simulink model "Solar_Tracker_Model_Dual_axis"  (R2024a)
settings: Solver=ode45  StartTime=0.0  StopTime=24  MaxStep=0.01  RelTol=1e-3
PreLoadFcn:
  | addpath(fullfile('WormAndGearConstraintSupport','Data'));
  | addpath(fullfile('WormAndGearConstraintSupport','Scripts'));
model workspace: external: MATLAB File WormAndGearConstraintParameters.m (data not in the file)
undefined symbols (not defined in the file): X, Y, Z
libraries: fl_lib x42, nesl_utility x18, WormAndGearConstraintLibrary x18, fl_ps_legacy_lib x17, sm_lib x9, ee_lib x4, simulink x2, SignalEditorBlockLib x2
(part 1 of 2)
CloseFcn:
  | rmpath(fullfile('WormAndGearConstraintSupport','Data'));
  | rmpath(fullfile('WormAndGearConstraintSupport','Scripts'));
Description:
  | Accurately sets up the solar panel according to the Sun's position
  | Project Name: Solar Tracker
  | Author: Kanak Sharma
  | Email: kanak.sharma1031@gmail.com
  | Date: 2024-06-25
  | License: This project is licensed under the MIT License - see the LICENSE file for details.
settings Model: Creator=The MathWorks, Inc.  LastModifiedBy=AADIL MALIK
settings SolverCC: AlgebraicLoopSolver=TrustRegion
settings DataIOCC: ReturnWorkspaceOutputs=off
settings OptimizationCC: ReuseModelBlockBuffer=off
settings DebuggingCC: UnconnectedInputMsg=warning  UnconnectedOutputMsg=warning  UnconnectedLineMsg=warning  SubsystemReferenceDiagnosticForUnitTest=warning  ArithmeticOperatorsInVariantConditions=warning
settings ModelReferenceCC: EnableRefExpFcnMdlSchedulingChecks=on
settings SFSimCC: SimUseLocalCustomCode=off  CustomCodeUndefinedFunction=UseInterfaceOnly
settings RTWCC: RTWUseLocalCustomCode=off  GPUComputeCapability=3.5
settings CodeAppCC: StateflowObjectComments=on
settings ConfigComp: CovMetricSettings=dswe
settings SimscapeCC: ExplicitSolverDiagnosticOptions=none  SimscapeNormalizeSystem=off  SimscapeNominalValues="[{\"value\":\"10\",\"unit\":\"V\"},{\"value\":\"1\",\"unit\":\"A\"},{\"value\":\"10\",\"unit\":\"N*m\"},{\"value\":\"10\",\"unit\":\"bar\"},{\"value\":\"100\",\"unit\":\"kJ/kg\"},{\"value\":\"1\",\"unit\":\"kW\"},{\"value\":\"300\",\"unit\":\"K\"},{\"value\":\"100\",\"unit\":\"cm^3/s\"},{\"value\":\"1\",\"unit\":\"kN\"},{\"value\":\"1\",\"unit\":\"g/cm^3\"},{\"value\":\"1\",\"unit\":\"l\"},{\"value\":\"1\",\"unit\":\"cm^2\"},{\"value\":\"60\",\"unit\":\"Hz\"}]"  SimscapeLogType=all  SimscapeLogSimulationStatistics=on  SimscapeLogName=simlogWormAndGearConstraint
settings DiagnosticsConfigSet: SimMechanicsUnconnectedFramePorts=none
settings ExplorerConfigSet: InternalSimMechanicsExplorerSettings="<ExplorerConfiguration><canonicalview>default</canonicalview><AnimationSetting><BasePlaybackSpeed>1.0</BasePlaybackSpeed><PlaybackSpeedFactor>1.0</PlaybackSpeedFactor></AnimationSetting><TilePanel><TileInfo><Tiles Columns=\"1\" Count=\"2\" Rows=\"2\"><Column Left=\"2\" Weight=\"1\"/><Column Left=\"959\" Weight=\"0.5003\"/><Row Top=\"2\" Weight=\"0.499\"/><Row Top=\"438\" Weight=\"0.501\"/><Row Top=\"875\"/><Tile Height=\"1\" Width=\"1\" X=\"0\" Y=\"0\"/><Tile Height=\"1\" Width=\"1\" X=\"0\" Y=\"1\"/></Tiles></TileInfo><SceneInfo><SceneViewer><BGColor><R>0.60000002384185791</R><G>0.60000002384185791</G><B>0.60000002384185791</B></BGColor><Camera><DoPerspective>off</DoPerspective><Position><X>1.5722270375482781</X><Y>0.036026125950558319</Y><Z>2.5132450829803226</Z></Position><Center><X>0.030597625568977493</X><Y>1.5776555379298589</Y><Z>0.97161567100102131</Z></Center><Up><X>-0.40824829046386307</X><Y>0.40824829046386307</Y><Z>0.81649658092772615</Z></Up><ViewLimDist>1</ViewLimDist><YLim>1.5517509961128235</YLim><XLim>3.445105256006924</XLim></Camera></SceneViewer><SceneViewer><BGColor><R>0.60000002384185791</R><G>0.60000002384185791</G><B>0.60000002384185791</B></BGColor><Camera><DoPerspective>on</DoPerspective><Position><X>0.052898448769590822</X><Y>3.2815089600888423</Y><Z>1.0106868675116196</Z></Position><Center><X>-0.01109217435380673</X><Y>3.0487464713239714</Y><Z>0.94979470185928261</Z></Center><Up><X>-0.054323829999052796</X><Y>-0.23871114009518463</Y><Z>0.96956996296744424</Z></Up><ViewLimDist>1</ViewLimDist><YLim>0.46630765815499858</YLim><XLim>1.0328496727358381</XLim></Camera></SceneViewer></SceneInfo></TilePanel><MechEditorPanel><Cameras><Camera><Id>Camera1</Id><Value><Name>Slew Drive View</Name><NativeCamera><PositionKeyframeSet><Keyframe><Time>+0.0000000000000000e+00</Time><Value><X>+5.2898448769590822e-02</X><Y>+3.2815089600888423e+00</Y><Z>+1.0106868675116196e+00</Z></Value></Keyframe></PositionKeyframeSet><CenterKeyframeSet><Keyframe><Time>+0.0000000000000000e+00</Time><Value><X>-1.1092174353806730e-02</X><Y>+3.0487464713239714e+00</Y><Z>+9.4979470185928261e-01</Z></Value></Keyframe></CenterKeyframeSet><UpVectorKeyframeSet><Keyframe><Time>+0.0000000000000000e+00</Time><Value><X>-5.4323829999052796e-02</X><Y>-2.3871114009518463e-01</Y><Z>+9.6956996296744424e-01</Z></Value></Keyframe></UpVectorKeyframeSet></NativeCamera></Value></Camera></Cameras><GfxPanelCameraMap><MapElement CameraMLId=\"Camera1\" GfxPanelIndex=\"1\"/></GfxPanelCameraMap><VideoCreator><PlaybackSpeedRatio>1.0</PlaybackSpeedRatio><FrameRate>30</FrameRate><VideoFormat>Motion JPEG AVI</VideoFormat><FrameSize>auto</FrameSize></VideoCreator></MechEditorPanel></ExplorerConfiguration>"

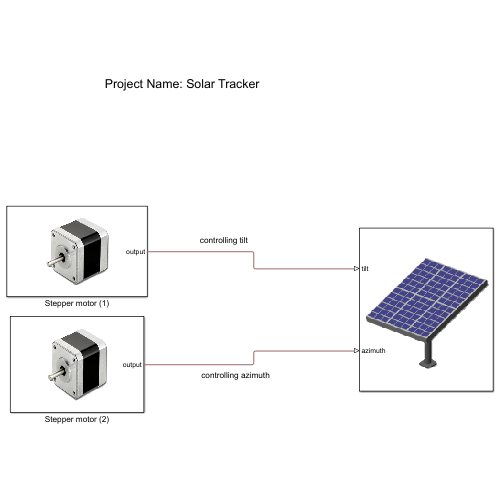
[thumbnail: Simulink's stored preview of the top-level diagram]
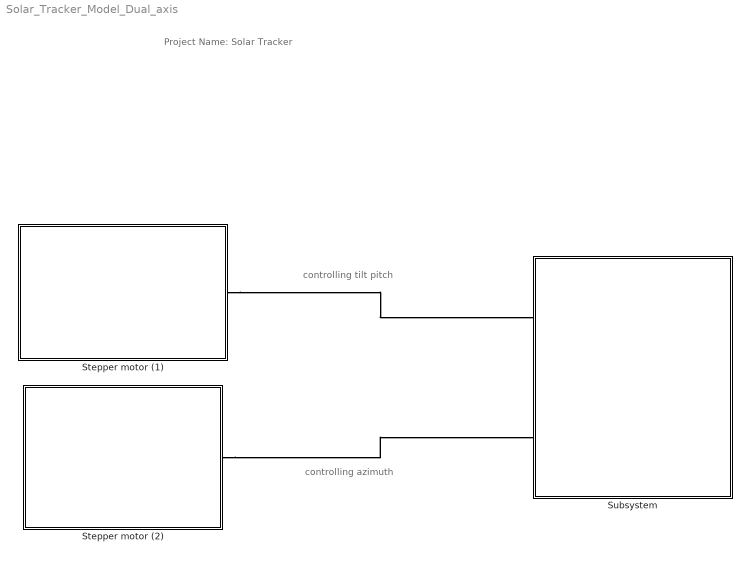
== system Solar_Tracker_Model_Dual_axis ==
  note: controlling azimuth
  note: controlling tilt pitch
  note: Project Name: Solar Tracker
  Stepper motor (1) : Subsystem
      mask Display: image('stepper_motor.jpg');
  Stepper motor (2) : Subsystem
      mask Display: image('stepper_motor.jpg');
  Subsystem : Subsystem
      mask Display: image('SolarTracker.png');
  connections:
  Stepper motor (1)/RConn1 -- Subsystem/LConn1
  Stepper motor (2)/RConn1 -- Subsystem/LConn2

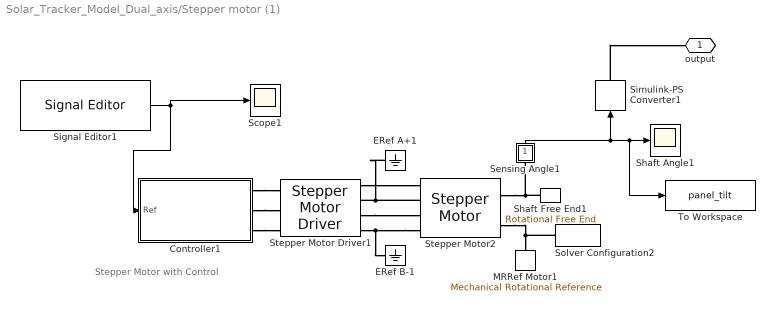
== system Solar_Tracker_Model_Dual_axis/Stepper motor (1) ==
  note: Stepper Motor with Control
  Controller1 : Subsystem  Variant=on  VariantControlMode=label  LabelModeActiveChoice=Position
      settings: AttributesFormatString=%<BlockChoice>
  ERef A+1 : fl_lib/Electrical/Electrical Elements/Electrical Reference
  ERef B-1 : fl_lib/Electrical/Electrical Elements/Electrical Reference
  MRRef Motor1 : fl_lib/Mechanical/Rotational Elements/Mechanical Rotational Reference
  Scope1 : Scope
  Sensing Angle1 : Subsystem
      mask Display: disp('a')
  Shaft Angle1 : Scope
  Shaft Free End1 : fl_lib/Mechanical/Rotational Elements/Rotational Free End  w_specify=off  w_priority=None  w=0 rad/s  w_nominal_specify=off  w_nominal_value=1  w_nominal_unit=rad/s
  Signal Editor1 : SignalEditorBlockLib/Signal Editor  FileName=elevation_signal_data.mat  ActiveScenario=dataset  ActiveSignal=elevation_signal_data  IsBus=off  OutputBusObjectStr=Bus: BusObject  SampleTime=0  Interpolate=off  ZeroCross=off  OutputAfterFinalValue=Setting to zero  Unit=inherit  PreserveSignalName=on  ApplySigPropsToAllScenarios=on  ApplySigPropsToAllSignals=off
  Simulink-PS Converter1 : nesl_utility/Simulink-PS Converter  PhysicalDomain=network_engine_domain  SubClassName=ps_input  LeftPortType=input  RightPortType=output  PseudoPeriodic=off  Frequencies=[]  NoiseDistribution=none  NoiseParameters=[]  Unit=deg  AffineConversion=off  FilteringAndDerivatives=filter  SimscapeFilterOrder=2  InputFilterTimeConstant=yawsignal.t_c  UdotUserProvided=1
  Solver Configuration2 : nesl_utility/Solver Configuration  PhysicalDomain=network_engine_domain  SubClassName=solver  LeftPortType=input  RightPortType=generic  Tones=[]  Harmonics=[]  SimulateNoise=off  Profile=off  UseLocalSampling=off  EnableSwitchedLinearOptims=on  FrequencyDomain=off  UseCCode=off  RelTol=0.001  AbsTol=1e-06  MinStep=1e-09  ToWorkspace=off  RevertToSquareIcSolve=off  NumHomotopyIterations=100  PhasorMode=off  PhasorModeNumHarmonics=1  ConsistencySolver=NEWTON_FTOL  IndexReductionMethod=DerivativeReplacement  DoDC=off  ResidualTolerance=1e-9  ConsistencyTolSource=GLOBAL  ConsistencyAbsTol=0.001  ConsistencyRelTol=0.001  ConsistencyTolFactor=0.001  UseLocalSolver=off  LocalSolverChoice=NE_BACKWARD_EULER_ADVANCER  ResolveIndetEquations=on  FunctionEvalNumThread=1  LocalSolverSampleTime=.001  DoFixedCost=off  MaxNonlinIter=3  MaxModeIter=2  ComputeImpulses=off  ImpulseIterations=2  LinearAlgebra=auto  LinearAlgebraNumThread=0  EquationFormulation=NE_TIME_EF  DelaysMemoryBudget=1024  AutomaticFiltering=on  FilteringTimeConstant=0.001  PartitionStorageMethod=AS_NEEDED  PartitionMemoryBudget=1024  PartitionMethod=FAST  MultibodyUseLocalSolver=off  MultibodyLocalSolverChoice=ODE1  MultibodyLocalSolverSampleTime=0.001
  Stepper Motor Driver1 : ee_lib/Electromechanical/Reluctance & Stepper/Stepper Motor Driver  step_or_av=1  step_rate_per_volt=10 Hz/V  Venable=2.5 V  Vreverse=2.5 V  supply_ports=ee.enum.supply_ports.hidesupply  Vm=5 V  Vsupply=10 V  half_stepping=0  stepping_mode=ee.enum.electromech.steppingMode.fullStep  numMicroSteps=4  Im=1.2 A
      settings: InternalSimscapePortConfiguration="{\"Bottom\":[],\"Left\":[{\"id\":\"ENA\",\"label\":\"ENA\",\"type\":\"foundation.electrical.electrical\"},{\"id\":\"REF\",\"label\":\"REF\",\"type\":\"foundation.electrical.electrical\"},{\"id\":\"REV\",\"label\":\"REV\",\"type\":\"foundation.electrical.electrical\"}],\"Right\":[{\"id\":\"pA\",\"label\":\"A+\",\"type\":\"foundation.electrical.electrical\"},{\"id\":\"nA\",\"label\":\"A-\",\"type\":\"foundation.electrical.electrical\"},{\"id\":\"pB\",\"label\":\"B+\",\"type\":\"foundation.electrical.electrical\"},{\"id\":\"nB\",\"label\":\"B-\",\"type\":\"foundation.electrical.electrical\"}],\"Top\":[]}"
  Stepper Motor2 : ee_lib/Electromechanical/Reluctance & Stepper/Stepper Motor  step_or_av=1  Ra=0.55 Ohm  La=0.0015 H  Km=0.19 N*m/A  Td=0 N*m  Rm=Inf Ohm  w_vec=[ 0 1000 3e+3 ] rpm  T_vec=[ 2 2 1 ] N*m  assert_if_slipping=0  J_total=1e-4 kg*m^2  max_step_rate=10 Hz  Step=1.8 deg  J=4.5e-05 kg*m^2  B=1e-02 N*m/(rad/s)  speed0=0 rpm  theta0=0 deg  alpha=[.00393, .00393] 1/K  Tmeas=25 degC  Tmeas2=125 degC  T_vec2=[1.7, 1.7, .85] N*m  half_stepping=ee.enum.electromech.steppingModeAveraged.fullStep  thermal_masses=[100, 100] J/K  initial_temperatures=[25, 25] degC  rotor_thermal_mass=50 J/K  rotor_initial_temperature=25 degC  Rm_percent_rotor=90
      settings: InternalSimscapePortConfiguration="{\"Bottom\":[],\"Left\":[{\"id\":\"pA\",\"label\":\"A+\",\"type\":\"foundation.electrical.electrical\"},{\"id\":\"nA\",\"label\":\"A-\",\"type\":\"foundation.electrical.electrical\"},{\"id\":\"pB\",\"label\":\"B+\",\"type\":\"foundation.electrical.electrical\"},{\"id\":\"nB\",\"label\":\"B-\",\"type\":\"foundation.electrical.electrical\"}],\"Right\":[{\"id\":\"R\",\"label\":\"R\",\"type\":\"foundation.mechanical.rotational.rotational\"},{\"id\":\"C\",\"label\":\"C\",\"type\":\"foundation.mechanical.rotational.rotational\"}],\"Top\":[]}"
  To Workspace : ToWorkspace  VariableName=panel_tilt  SampleTime=-1
  output : PMIOPort  Side=Right
  wires:
  Signal Editor1/1 -> Scope1/1, Controller1/1(Ref)
  Sensing Angle1/1(theta) -> Simulink-PS Converter1/1, To Workspace/1, Shaft Angle1/1
  connections:
  Stepper Motor2/LConn4 -- Stepper Motor Driver1/RConn4 -- ERef B-1/LConn1
  Stepper Motor Driver1/RConn3 -- Stepper Motor2/LConn3
  Solver Configuration2/RConn1 -- Stepper Motor2/RConn2 -- MRRef Motor1/LConn1
  Shaft Free End1/LConn1 -- Stepper Motor2/RConn1 -- Sensing Angle1/LConn1
  Controller1/RConn3 -- Stepper Motor Driver1/LConn3
  Controller1/RConn1 -- Stepper Motor Driver1/LConn1
  Controller1/RConn2 -- Stepper Motor Driver1/LConn2
  Simulink-PS Converter1/RConn1 -- output/RConn1
  ERef A+1/LConn1 -- Stepper Motor2/LConn2 -- Stepper Motor Driver1/RConn2
  Stepper Motor Driver1/RConn1 -- Stepper Motor2/LConn1

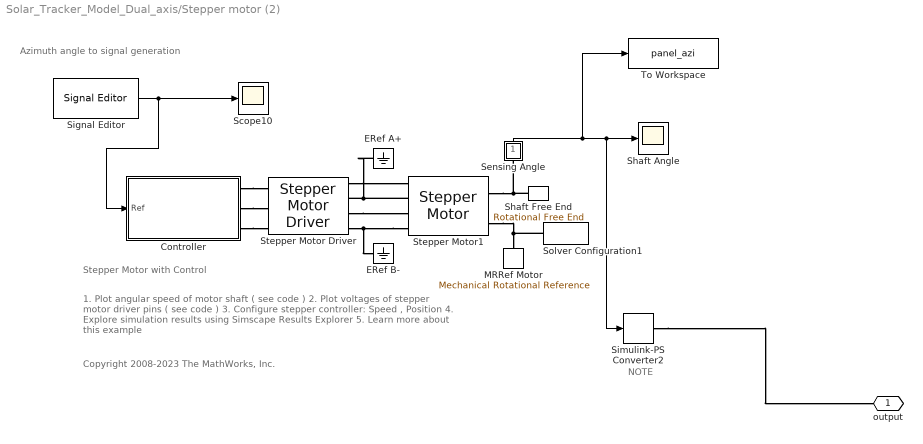
== system Solar_Tracker_Model_Dual_axis/Stepper motor (2) ==
  note: NOTE
  note: Stepper Motor with Control
  note: 1. Plot angular speed of motor shaft ( see code )
      | 2. Plot voltages of stepper motor driver pins ( see code )
      | 3. Configure stepper controller: Speed , Position
      | 4. Explore simulation results using Simscape Results Explorer
      | 5. Learn more about this example
  note: Azimuth angle to signal generation
  note: Copyright 2008-2023 The MathWorks, Inc.
  Controller : Subsystem  Variant=on  VariantControlMode=label  LabelModeActiveChoice=Position
      settings: AttributesFormatString=%<BlockChoice>
  ERef A+ : fl_lib/Electrical/Electrical Elements/Electrical Reference
  ERef B- : fl_lib/Electrical/Electrical Elements/Electrical Reference
  MRRef Motor : fl_lib/Mechanical/Rotational Elements/Mechanical Rotational Reference
  Scope10 : Scope
  Sensing Angle : Subsystem
      mask Display: disp('a')
  Shaft Angle : Scope
  Shaft Free End : fl_lib/Mechanical/Rotational Elements/Rotational Free End  w_specify=off  w_priority=None  w=0 rad/s  w_nominal_specify=off  w_nominal_value=1  w_nominal_unit=rad/s
  Signal Editor : SignalEditorBlockLib/Signal Editor  FileName=azimuth_signal_data.mat  ActiveScenario=dataset  ActiveSignal=azimuth_signal_data  IsBus=off  OutputBusObjectStr=Bus: BusObject  SampleTime=0  Interpolate=off  ZeroCross=off  OutputAfterFinalValue=Setting to zero  Unit=inherit  PreserveSignalName=on  ApplySigPropsToAllScenarios=on  ApplySigPropsToAllSignals=off
  Simulink-PS Converter2 : nesl_utility/Simulink-PS Converter  PhysicalDomain=network_engine_domain  SubClassName=ps_input  LeftPortType=input  RightPortType=output  PseudoPeriodic=off  Frequencies=[]  NoiseDistribution=none  NoiseParameters=[]  Unit=deg  AffineConversion=off  FilteringAndDerivatives=filter  SimscapeFilterOrder=2  InputFilterTimeConstant=yawsignal.t_c  UdotUserProvided=1
  Solver Configuration1 : nesl_utility/Solver Configuration  PhysicalDomain=network_engine_domain  SubClassName=solver  LeftPortType=input  RightPortType=generic  Tones=[]  Harmonics=[]  SimulateNoise=off  Profile=off  UseLocalSampling=off  EnableSwitchedLinearOptims=on  FrequencyDomain=off  UseCCode=off  RelTol=0.001  AbsTol=1e-06  MinStep=1e-09  ToWorkspace=off  RevertToSquareIcSolve=off  NumHomotopyIterations=100  PhasorMode=off  PhasorModeNumHarmonics=1  ConsistencySolver=NEWTON_FTOL  IndexReductionMethod=DerivativeReplacement  DoDC=off  ResidualTolerance=1e-9  ConsistencyTolSource=GLOBAL  ConsistencyAbsTol=0.001  ConsistencyRelTol=0.001  ConsistencyTolFactor=0.001  UseLocalSolver=off  LocalSolverChoice=NE_BACKWARD_EULER_ADVANCER  ResolveIndetEquations=on  FunctionEvalNumThread=1  LocalSolverSampleTime=.001  DoFixedCost=off  MaxNonlinIter=3  MaxModeIter=2  ComputeImpulses=off  ImpulseIterations=2  LinearAlgebra=auto  LinearAlgebraNumThread=0  EquationFormulation=NE_TIME_EF  DelaysMemoryBudget=1024  AutomaticFiltering=on  FilteringTimeConstant=0.001  PartitionStorageMethod=AS_NEEDED  PartitionMemoryBudget=1024  PartitionMethod=FAST  MultibodyUseLocalSolver=off  MultibodyLocalSolverChoice=ODE1  MultibodyLocalSolverSampleTime=0.001
  Stepper Motor Driver : ee_lib/Electromechanical/Reluctance & Stepper/Stepper Motor Driver  step_or_av=1  step_rate_per_volt=10 Hz/V  Venable=2.5 V  Vreverse=2.5 V  supply_ports=ee.enum.supply_ports.hidesupply  Vm=5 V  Vsupply=10 V  half_stepping=0  stepping_mode=ee.enum.electromech.steppingMode.fullStep  numMicroSteps=4  Im=1.2 A
      settings: InternalSimscapePortConfiguration="{\"Bottom\":[],\"Left\":[{\"id\":\"ENA\",\"label\":\"ENA\",\"type\":\"foundation.electrical.electrical\"},{\"id\":\"REF\",\"label\":\"REF\",\"type\":\"foundation.electrical.electrical\"},{\"id\":\"REV\",\"label\":\"REV\",\"type\":\"foundation.electrical.electrical\"}],\"Right\":[{\"id\":\"pA\",\"label\":\"A+\",\"type\":\"foundation.electrical.electrical\"},{\"id\":\"nA\",\"label\":\"A-\",\"type\":\"foundation.electrical.electrical\"},{\"id\":\"pB\",\"label\":\"B+\",\"type\":\"foundation.electrical.electrical\"},{\"id\":\"nB\",\"label\":\"B-\",\"type\":\"foundation.electrical.electrical\"}],\"Top\":[]}"
  Stepper Motor1 : ee_lib/Electromechanical/Reluctance & Stepper/Stepper Motor  step_or_av=1  Ra=0.55 Ohm  La=0.0015 H  Km=0.19 N*m/A  Td=0 N*m  Rm=Inf Ohm  w_vec=[ 0 1000 3e+3 ] rpm  T_vec=[ 2 2 1 ] N*m  assert_if_slipping=0  J_total=1e-4 kg*m^2  max_step_rate=10 Hz  Step=1.8 deg  J=4.5e-05 kg*m^2  B=1e-02 N*m/(rad/s)  speed0=0 rpm  theta0=0 deg  alpha=[.00393, .00393] 1/K  Tmeas=25 degC  Tmeas2=125 degC  T_vec2=[1.7, 1.7, .85] N*m  half_stepping=ee.enum.electromech.steppingModeAveraged.fullStep  thermal_masses=[100, 100] J/K  initial_temperatures=[25, 25] degC  rotor_thermal_mass=50 J/K  rotor_initial_temperature=25 degC  Rm_percent_rotor=90
      settings: InternalSimscapePortConfiguration="{\"Bottom\":[],\"Left\":[{\"id\":\"pA\",\"label\":\"A+\",\"type\":\"foundation.electrical.electrical\"},{\"id\":\"nA\",\"label\":\"A-\",\"type\":\"foundation.electrical.electrical\"},{\"id\":\"pB\",\"label\":\"B+\",\"type\":\"foundation.electrical.electrical\"},{\"id\":\"nB\",\"label\":\"B-\",\"type\":\"foundation.electrical.electrical\"}],\"Right\":[{\"id\":\"R\",\"label\":\"R\",\"type\":\"foundation.mechanical.rotational.rotational\"},{\"id\":\"C\",\"label\":\"C\",\"type\":\"foundation.mechanical.rotational.rotational\"}],\"Top\":[]}"
  To Workspace : ToWorkspace  VariableName=panel_azi  SampleTime=-1
  output : PMIOPort  Side=Right
  wires:
  Sensing Angle/1(theta) -> To Workspace/1, Simulink-PS Converter2/1, Shaft Angle/1
  Signal Editor/1 -> Controller/1(Ref), Scope10/1
  connections:
  Controller/RConn2 -- Stepper Motor Driver/LConn2
  Stepper Motor1/LConn4 -- Stepper Motor Driver/RConn4 -- ERef B-/LConn1
  Solver Configuration1/RConn1 -- Stepper Motor1/RConn2 -- MRRef Motor/LConn1
  ERef A+/LConn1 -- Stepper Motor1/LConn2 -- Stepper Motor Driver/RConn2
  Shaft Free End/LConn1 -- Stepper Motor1/RConn1 -- Sensing Angle/LConn1
  Controller/RConn1 -- Stepper Motor Driver/LConn1
  Stepper Motor Driver/RConn3 -- Stepper Motor1/LConn3
  Controller/RConn3 -- Stepper Motor Driver/LConn3
  Stepper Motor Driver/RConn1 -- Stepper Motor1/LConn1
  Simulink-PS Converter2/RConn1 -- output/RConn1

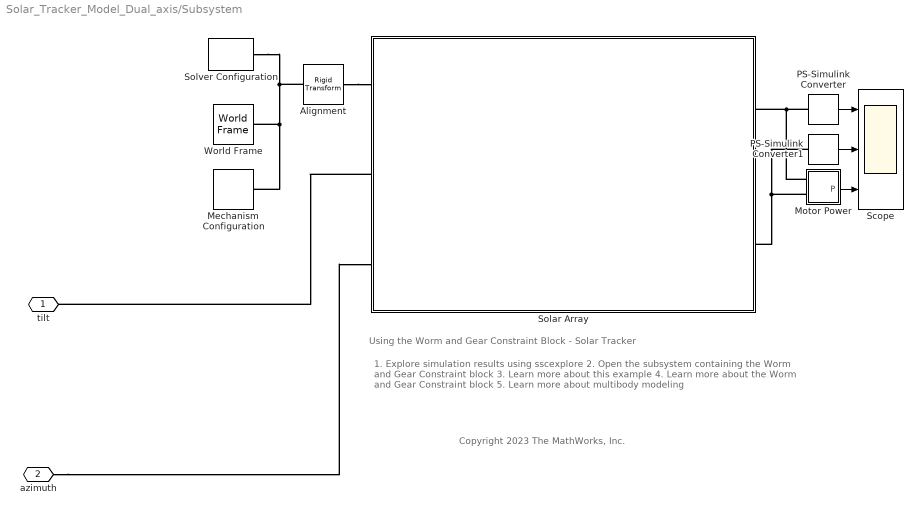
== system Solar_Tracker_Model_Dual_axis/Subsystem ==
  note: Copyright 2023 The MathWorks, Inc.
  note: Using the Worm and Gear Constraint Block - Solar Tracker
  note: 1. Explore simulation results using sscexplore
      | 2. Open the subsystem containing the Worm and Gear Constraint block
      | 3. Learn more about this example
      | 4. Learn more about the Worm and Gear Constraint block
      | 5. Learn more about multibody modeling
  Alignment : sm_lib/Frames and Transforms/Rigid Transform  RotationMethod=AlignedAxes  FollAlignAxisA=+Z  BaseAlignAxisA=+Z  FollAlignAxisB=+Y  BaseAlignAxisB=-X  RotationStandardAxis=+Z  RotationAngle=0.0  RotationAngleUnits=deg  RotationArbitraryAxis=[0 0 1]  RotationSequenceAxes=FollowerAxes  RotationSequence=XYX  RotationSequenceAngles=[0 0 0]  RotationSequenceAnglesUnits=deg  RotationMatrix=[1 0 0; 0 1 0; 0 0 1]  Quaternion=[1 0 0 0]  TranslationMethod=None  TranslationCartesianOffset=[0 0 0]  TranslationCartesianOffsetUnits=m  TranslationStandardAxis=+Z  TranslationStandardOffset=0  TranslationStandardOffsetUnits=m  TranslationROffset=0  TranslationROffsetUnits=m  TranslationThetaOffset=0  TranslationThetaOffsetUnits=deg  TranslationZOffset=0  TranslationZOffsetUnits=m
  Mechanism Configuration : sm_lib/Utilities/Mechanism Configuration  UniformGravity=Constant  GravityVector=[0 0 -9.80665]  GravityVectorUnits=m/s^2  LinearizationDelta=0.001  JointModeTransitionNonlinearIterations=2
  Motor Power : Subsystem
  PS-Simulink Converter : nesl_utility/PS-Simulink Converter  PhysicalDomain=network_engine_domain  SubClassName=ps_output  LeftPortType=input  RightPortType=output  PseudoPeriodic=off  Frequencies=[]  VectorFormat=1-D array  Unit=deg/s  AffineConversion=off
  PS-Simulink Converter1 : nesl_utility/PS-Simulink Converter  PhysicalDomain=network_engine_domain  SubClassName=ps_output  LeftPortType=input  RightPortType=output  PseudoPeriodic=off  Frequencies=[]  VectorFormat=1-D array  Unit=N*m  AffineConversion=off
  Scope : Scope  NumInputPorts=3
  Solar Array : Subsystem
      mask Display:
      | image(fullfile('WormAndGearConstraintSupport','Images','SolarArray.png'));
      | port_label('lconn',1,'W');
      | port_label('lconn',2,'yaw');
      | port_label('lconn',3,'pitch');
      | port_label('rconn',1,'wWorm');
      | port_label('rconn',2,'tWorm');
  Solver Configuration : nesl_utility/Solver Configuration  PhysicalDomain=network_engine_domain  SubClassName=solver  LeftPortType=input  RightPortType=generic  Tones=[]  Harmonics=[]  SimulateNoise=off  Profile=off  UseLocalSampling=off  EnableSwitchedLinearOptims=on  FrequencyDomain=off  UseCCode=off  RelTol=0.001  AbsTol=1e-06  MinStep=1e-09  ToWorkspace=off  RevertToSquareIcSolve=off  NumHomotopyIterations=100  PhasorMode=off  PhasorModeNumHarmonics=1  ConsistencySolver=NEWTON_FTOL  IndexReductionMethod=DerivativeReplacement  DoDC=off  ResidualTolerance=1e-09  ConsistencyTolSource=GLOBAL  ConsistencyAbsTol=0.001  ConsistencyRelTol=0.001  ConsistencyTolFactor=0.001  UseLocalSolver=off  LocalSolverChoice=NE_BACKWARD_EULER_ADVANCER  ResolveIndetEquations=on  FunctionEvalNumThread=1  LocalSolverSampleTime=0.001  DoFixedCost=off  MaxNonlinIter=3  MaxModeIter=2  ComputeImpulses=off  ImpulseIterations=2  LinearAlgebra=Sparse  LinearAlgebraNumThread=0  EquationFormulation=NE_TIME_EF  DelaysMemoryBudget=1024  AutomaticFiltering=on  FilteringTimeConstant=0.001  PartitionStorageMethod=AS_NEEDED  PartitionMemoryBudget=1024  PartitionMethod=FAST  MultibodyUseLocalSolver=off  MultibodyLocalSolverChoice=ODE1  MultibodyLocalSolverSampleTime=0.001
  World Frame : sm_lib/Frames and Transforms/World Frame
  tilt : PMIOPort  Side=Left
  azimuth : PMIOPort  Port=2  Side=Left
  wires:
  PS-Simulink Converter1/1 -> Scope/2
  Motor Power/1(P) -> Scope/3
  PS-Simulink Converter/1 -> Scope/1
  connections:
  PS-Simulink Converter/LConn1 -- Motor Power/LConn1 -- Solar Array/RConn1
  World Frame/RConn1 -- Solver Configuration/RConn1 -- Alignment/LConn1 -- Mechanism Configuration/RConn1
  Alignment/RConn1 -- Solar Array/LConn1
  PS-Simulink Converter1/LConn1 -- Motor Power/LConn2 -- Solar Array/RConn2
  azimuth/RConn1 -- Solar Array/LConn3
  Solar Array/LConn2 -- tilt/RConn1

== system Solar_Tracker_Model_Dual_axis/Stepper motor (1)/Controller1 ==
  Ref : Inport
  Position : Subsystem  VariantControl=Position
  Speed : Subsystem  VariantControl=Speed
  PWM : PMIOPort  Side=Right
  0v : PMIOPort  Port=2  Side=Right
  REV : PMIOPort  Port=3  Side=Right

== system Solar_Tracker_Model_Dual_axis/Stepper motor (1)/Sensing Angle1 ==
  MRRef : fl_lib/Mechanical/Rotational Elements/Mechanical Rotational Reference
  Motion Sensor : fl_lib/Mechanical/Mechanical Sensors/Ideal Rotational Motion Sensor  reference=foundation.enum.MeasurementReference.difference  acceleration_port=false  velocity_port=true  position_port=true  wrap_angle=simscape.enum.onoff.off  offset=0 rad
  deg : nesl_utility/PS-Simulink Converter  PhysicalDomain=network_engine_domain  SubClassName=ps_output  LeftPortType=input  RightPortType=output  PseudoPeriodic=off  Frequencies=[]  VectorFormat=1-D array  Unit=deg  AffineConversion=off
  R : PMIOPort  Side=Left
  theta : Outport  VectorParamsAs1DForOutWhenUnconnected=off
  wires:
  deg/1 -> theta/1
  connections:
  R/RConn1 -- Motion Sensor/LConn1
  Motion Sensor/RConn3 -- deg/LConn1
  MRRef/LConn1 -- Motion Sensor/RConn1

== system Solar_Tracker_Model_Dual_axis/Stepper motor (2)/Controller ==
  Ref : Inport
  Position : Subsystem  VariantControl=Position
  Speed : Subsystem  VariantControl=Speed
  PWM : PMIOPort  Side=Right
  0v : PMIOPort  Port=2  Side=Right
  REV : PMIOPort  Port=3  Side=Right

== system Solar_Tracker_Model_Dual_axis/Stepper motor (2)/Sensing Angle ==
  MRRef : fl_lib/Mechanical/Rotational Elements/Mechanical Rotational Reference
  Motion Sensor : fl_lib/Mechanical/Mechanical Sensors/Ideal Rotational Motion Sensor  reference=foundation.enum.MeasurementReference.difference  acceleration_port=false  velocity_port=true  position_port=true  wrap_angle=simscape.enum.onoff.off  offset=0 rad
  deg : nesl_utility/PS-Simulink Converter  PhysicalDomain=network_engine_domain  SubClassName=ps_output  LeftPortType=input  RightPortType=output  PseudoPeriodic=off  Frequencies=[]  VectorFormat=1-D array  Unit=deg  AffineConversion=off
  R : PMIOPort  Side=Left
  theta : Outport  VectorParamsAs1DForOutWhenUnconnected=off
  wires:
  deg/1 -> theta/1
  connections:
  R/RConn1 -- Motion Sensor/LConn1
  Motion Sensor/RConn3 -- deg/LConn1
  MRRef/LConn1 -- Motion Sensor/RConn1

== system Solar_Tracker_Model_Dual_axis/Subsystem/Motor Power ==
  Motor Power : fl_ps_legacy_lib/Legacy Physical Signals/Functions/PS Product
  PS-Simulink Converter2 : nesl_utility/PS-Simulink Converter  PhysicalDomain=network_engine_domain  SubClassName=ps_output  LeftPortType=input  RightPortType=output  PseudoPeriodic=off  Frequencies=[]  VectorFormat=1-D array  Unit=kW  AffineConversion=off
  w : PMIOPort  Side=Left
  t : PMIOPort  Port=2  Side=Left
  P : Outport
  wires:
  PS-Simulink Converter2/1 -> P/1
  connections:
  PS-Simulink Converter2/LConn1 -- Motor Power/RConn1
  Motor Power/LConn2 -- t/RConn1
  Motor Power/LConn1 -- w/RConn1

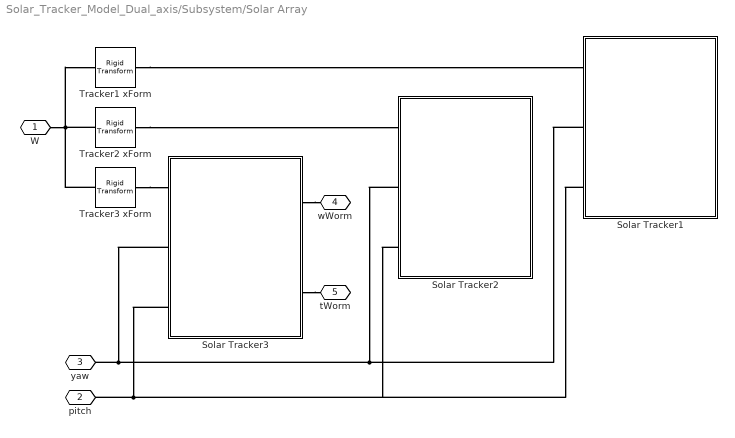
== system Solar_Tracker_Model_Dual_axis/Subsystem/Solar Array ==
  Solar Tracker1 : Subsystem
      mask Display:
      | image(fullfile('WormAndGearConstraintSupport','Images','SolarTracker.png'));
      | port_label('lconn',1,'B');
      | port_label('lconn',2,'y');
      | port_label('lconn',3,'p');
  Solar Tracker2 : Subsystem
      mask Display:
      | image(fullfile('WormAndGearConstraintSupport','Images','SolarTracker.png'));
      | port_label('lconn',1,'B');
      | port_label('lconn',2,'y');
      | port_label('lconn',3,'p');
  Solar Tracker3 : Subsystem
      mask Display:
      | image(fullfile('WormAndGearConstraintSupport','Images','SolarTracker.png'));
      | port_label('lconn',1,'B');
      | port_label('lconn',2,'y');
      | port_label('lconn',3,'p');
      | port_label('rconn',1,'w');
      | port_label('rconn',2,'t');
  Tracker1 xForm : sm_lib/Frames and Transforms/Rigid Transform  RotationMethod=None  FollAlignAxisA=+X  BaseAlignAxisA=+Y  FollAlignAxisB=+Y  BaseAlignAxisB=+Z  RotationStandardAxis=+Z  RotationAngle=0.0  RotationAngleUnits=deg  RotationArbitraryAxis=[0 0 1]  RotationSequenceAxes=FollowerAxes  RotationSequence=XYX  RotationSequenceAngles=[0 0 0]  RotationSequenceAnglesUnits=deg  RotationMatrix=[1 0 0; 0 1 0; 0 0 1]  Quaternion=[1 0 0 0]  TranslationMethod=Cartesian  TranslationCartesianOffset=tracker1_offset  TranslationCartesianOffsetUnits=m  TranslationStandardAxis=+Z  TranslationStandardOffset=0  TranslationStandardOffsetUnits=m  TranslationROffset=0  TranslationROffsetUnits=m  TranslationThetaOffset=0  TranslationThetaOffsetUnits=deg  TranslationZOffset=0  TranslationZOffsetUnits=m
  Tracker2 xForm : sm_lib/Frames and Transforms/Rigid Transform  RotationMethod=None  FollAlignAxisA=+Z  BaseAlignAxisA=+Z  FollAlignAxisB=+Y  BaseAlignAxisB=-X  RotationStandardAxis=+Z  RotationAngle=0.0  RotationAngleUnits=deg  RotationArbitraryAxis=[0 0 1]  RotationSequenceAxes=FollowerAxes  RotationSequence=XYX  RotationSequenceAngles=[0 0 0]  RotationSequenceAnglesUnits=deg  RotationMatrix=[1 0 0; 0 1 0; 0 0 1]  Quaternion=[1 0 0 0]  TranslationMethod=Cartesian  TranslationCartesianOffset=tracker2_offset  TranslationCartesianOffsetUnits=m  TranslationStandardAxis=+Z  TranslationStandardOffset=0  TranslationStandardOffsetUnits=m  TranslationROffset=0  TranslationROffsetUnits=m  TranslationThetaOffset=0  TranslationThetaOffsetUnits=deg  TranslationZOffset=0  TranslationZOffsetUnits=m
  Tracker3 xForm : sm_lib/Frames and Transforms/Rigid Transform  RotationMethod=None  FollAlignAxisA=+X  BaseAlignAxisA=+Y  FollAlignAxisB=+Y  BaseAlignAxisB=+Z  RotationStandardAxis=+Z  RotationAngle=0.0  RotationAngleUnits=deg  RotationArbitraryAxis=[0 0 1]  RotationSequenceAxes=FollowerAxes  RotationSequence=XYX  RotationSequenceAngles=[0 0 0]  RotationSequenceAnglesUnits=deg  RotationMatrix=[1 0 0; 0 1 0; 0 0 1]  Quaternion=[1 0 0 0]  TranslationMethod=Cartesian  TranslationCartesianOffset=tracker3_offset  TranslationCartesianOffsetUnits=m  TranslationStandardAxis=+Z  TranslationStandardOffset=0  TranslationStandardOffsetUnits=m  TranslationROffset=0  TranslationROffsetUnits=m  TranslationThetaOffset=0  TranslationThetaOffsetUnits=deg  TranslationZOffset=0  TranslationZOffsetUnits=m
  W : PMIOPort  Side=Left
  pitch : PMIOPort  Port=2  Side=Left
  yaw : PMIOPort  Port=3  Side=Left
  wWorm : PMIOPort  Port=4  Side=Right
  tWorm : PMIOPort  Port=5  Side=Right
  connections:
  Tracker3 xForm/LConn1 -- Tracker1 xForm/LConn1 -- W/RConn1 -- Tracker2 xForm/LConn1
  Tracker3 xForm/RConn1 -- Solar Tracker3/LConn1
  Solar Tracker3/RConn2 -- tWorm/RConn1
  Solar Tracker3/LConn3 -- Solar Tracker2/LConn3 -- Solar Tracker1/LConn3 -- pitch/RConn1
  Solar Tracker3/RConn1 -- wWorm/RConn1
  Solar Tracker2/LConn2 -- Solar Tracker1/LConn2 -- Solar Tracker3/LConn2 -- yaw/RConn1
  Tracker2 xForm/RConn1 -- Solar Tracker2/LConn1
  Tracker1 xForm/RConn1 -- Solar Tracker1/LConn1

== system Solar_Tracker_Model_Dual_axis/Stepper motor (1)/Controller1/Position ==
  Ref : Inport
  Algorithm and Pulse Generation : Subsystem
  ERef : fl_lib/Electrical/Electrical Elements/Electrical Reference
  PWM : PMIOPort  Side=Right
  0v : PMIOPort  Port=2  Side=Right
  REV : PMIOPort  Port=3  Side=Right
  wires:
  Ref/1 -> Algorithm and Pulse Generation/1(Reference)
  connections:
  Algorithm and Pulse Generation/RConn2 -- PWM/RConn1
  Algorithm and Pulse Generation/RConn1 -- REV/RConn1
  ERef/LConn1 -- 0v/RConn1

== system Solar_Tracker_Model_Dual_axis/Stepper motor (1)/Controller1/Speed ==
  note: Step rate and direction algorithm implemented on a microprocessor or dedicated discrete chip
  Ref : Inport
  ERef : fl_lib/Electrical/Electrical Elements/Electrical Reference
  Step Rate and Direction : Subsystem
  Voltage-Controlled Pulse Generator : Subsystem
  PWM : PMIOPort  Side=Right
  0v : PMIOPort  Port=2  Side=Right
  REV : PMIOPort  Port=3  Side=Right
  wires:
  Ref/1 -> Step Rate and Direction/1(Reference)
  connections:
  PWM/RConn1 -- Voltage-Controlled Pulse Generator/RConn1
  Voltage-Controlled Pulse Generator/RConn2 -- 0v/RConn1 -- ERef/LConn1
  Step Rate and Direction/RConn1 -- REV/RConn1
  Step Rate and Direction/RConn2 -- Voltage-Controlled Pulse Generator/LConn1

== system Solar_Tracker_Model_Dual_axis/Stepper motor (2)/Controller/Position ==
  Ref : Inport
  Algorithm and Pulse Generation : Subsystem
  ERef : fl_lib/Electrical/Electrical Elements/Electrical Reference
  PWM : PMIOPort  Side=Right
  0v : PMIOPort  Port=2  Side=Right
  REV : PMIOPort  Port=3  Side=Right
  wires:
  Ref/1 -> Algorithm and Pulse Generation/1(Reference)
  connections:
  Algorithm and Pulse Generation/RConn2 -- PWM/RConn1
  Algorithm and Pulse Generation/RConn1 -- REV/RConn1
  ERef/LConn1 -- 0v/RConn1

== system Solar_Tracker_Model_Dual_axis/Stepper motor (2)/Controller/Speed ==
  note: Step rate and direction algorithm implemented on a microprocessor or dedicated discrete chip
  Ref : Inport
  ERef : fl_lib/Electrical/Electrical Elements/Electrical Reference
  Step Rate and Direction : Subsystem
  Voltage-Controlled Pulse Generator : Subsystem
  PWM : PMIOPort  Side=Right
  0v : PMIOPort  Port=2  Side=Right
  REV : PMIOPort  Port=3  Side=Right
  wires:
  Ref/1 -> Step Rate and Direction/1(Reference)
  connections:
  PWM/RConn1 -- Voltage-Controlled Pulse Generator/RConn1
  Voltage-Controlled Pulse Generator/RConn2 -- 0v/RConn1 -- ERef/LConn1
  Step Rate and Direction/RConn1 -- REV/RConn1
  Step Rate and Direction/RConn2 -- Voltage-Controlled Pulse Generator/LConn1

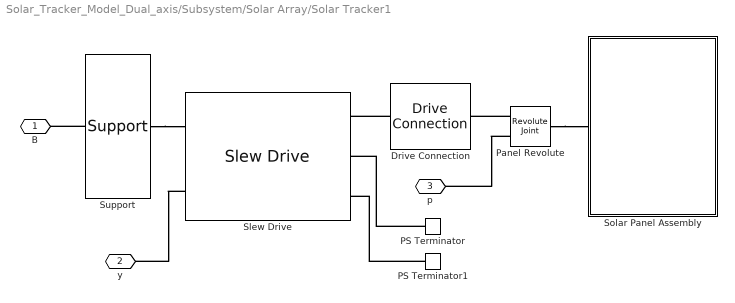
== system Solar_Tracker_Model_Dual_axis/Subsystem/Solar Array/Solar Tracker1 ==
  Drive Connection : WormAndGearConstraintLibrary/Drive Connection  connRadius=driveconn.connectionRadius  connThickness=driveconn.connectionThickness  connLength=driveconn.connectionLength  bracketWidth=driveconn.bracketWidthHeight  bracketThickness=driveconn.bracketThickness  holeRadius=driveconn.holeRadius  holeOffset=driveconn.holeOffset  baseThickness=driveconn.baseThickness  rho=driveconn.density  color=driveconn.color
      settings: LibrarySourceBlock=sm_solar_tracker_lib/Drive Connection
  PS Terminator : fl_lib/Physical Signals/Sinks/PS Terminator
  PS Terminator1 : fl_lib/Physical Signals/Sinks/PS Terminator
  Panel Revolute : sm_lib/Joints/Revolute Joint  JointMode=Normal  CompositeWrenchDir=FollowerOnBase  CompositeWrenchFrame=BaseFrame  SenseConstraintForce=off  SenseConstraintTorque=off  SenseTotalForce=off  SenseTotalTorque=off  PositionTargetSpecify=on  PositionTargetPriority=High  PositionTargetValue=panelrevolute.q0  PositionTargetValueUnits=deg  VelocityTargetSpecify=off  VelocityTargetPriority=High  VelocityTargetValue=0  VelocityTargetValueUnits=deg/s  EquilibriumPosition=0  EquilibriumPositionUnits=deg  SpringStiffness=0  SpringStiffnessUnits=N*m/deg  DampingCoefficient=0  DampingCoefficientUnits=N*m/(deg/s)  LowerLimitSpecify=off  LowerLimitBound=-90  LowerLimitBoundUnits=deg  LowerLimitStiffness=1e4  LowerLimitStiffnessUnits=N*m/deg  LowerLimitDamping=10  LowerLimitDampingUnits=N*m/(deg/s)  LowerLimitTransitionRegionWidth=0.1  LowerLimitTransitionRegionWidthUnits=deg  UpperLimitSpecify=off  UpperLimitBound=90  UpperLimitBoundUnits=deg  UpperLimitStiffness=1e4  UpperLimitStiffnessUnits=N*m/deg  UpperLimitDamping=10  UpperLimitDampingUnits=N*m/(deg/s)  UpperLimitTransitionRegionWidth=0.1  UpperLimitTransitionRegionWidthUnits=deg  TorqueActuationMode=ComputedTorque  MotionActuationMode=InputMotion  SensePosition=off  SenseVelocity=off  SenseAcceleration=off  SenseTorqueForce=off  SenseLowerLimitTorqueForce=off  SenseUpperLimitTorqueForce=off
  Slew Drive : WormAndGearConstraintLibrary/Slew Drive  wormLeadAngle=slewdrive.wormLeadAngle  wormLength=slewdrive.wormLength  gearOuterRadius=slewdrive.gearOuterRadius  gearInnerRadius=slewdrive.gearInnerRadius  gearExposedRadius=slewdrive.gearExposedRadius  ratio=slewdrive.ratio  housingThickness=slewdrive.housingThickness  bWormRevolute=slewdrive.wormRevoluteDamping  wormRho=slewdrive.wormDensity  gearRho=slewdrive.gearDensity  housingRho=slewdrive.housingDensity  wormColor=slewdrive.wormColor  gearColor=slewdrive.gearColor  housingColor=slewdrive.housingColor  housingOpacity=slewdrive.housingOpacity
      settings: LibrarySourceBlock=sm_solar_tracker_lib/Slew Drive
  Solar Panel Assembly : Subsystem
      mask Display:
      | image(fullfile('WormAndGearConstraintSupport','Images','SolarPanel.png'));
      | port_label('lconn',1,'H');
  Support : WormAndGearConstraintLibrary/Support  columnRadius=support.columnRadius  columnThickness=support.columnThickness  columnHeight=support.columnHeight  baseWidth=support.baseWidth  baseThickness=support.baseThickness  rho=support.density  color=support.color
      settings: LibrarySourceBlock=sm_solar_tracker_lib/Support
  B : PMIOPort  Side=Left
  y : PMIOPort  Port=2  Side=Left
  p : PMIOPort  Port=3  Side=Left
  connections:
  Support/LConn1 -- B/RConn1
  Support/RConn1 -- Slew Drive/LConn1
  Drive Connection/LConn1 -- Slew Drive/RConn1
  Panel Revolute/LConn1 -- Drive Connection/RConn1
  PS Terminator/LConn1 -- Slew Drive/RConn2
  Slew Drive/LConn2 -- y/RConn1
  Panel Revolute/LConn2 -- p/RConn1
  Panel Revolute/RConn1 -- Solar Panel Assembly/LConn1
  PS Terminator1/LConn1 -- Slew Drive/RConn3

== system Solar_Tracker_Model_Dual_axis/Subsystem/Solar Array/Solar Tracker2 ==
  Drive Connection : WormAndGearConstraintLibrary/Drive Connection  connRadius=driveconn.connectionRadius  connThickness=driveconn.connectionThickness  connLength=driveconn.connectionLength  bracketWidth=driveconn.bracketWidthHeight  bracketThickness=driveconn.bracketThickness  holeRadius=driveconn.holeRadius  holeOffset=driveconn.holeOffset  baseThickness=driveconn.baseThickness  rho=driveconn.density  color=driveconn.color
      settings: LibrarySourceBlock=sm_solar_tracker_lib/Drive Connection
  PS Terminator : fl_lib/Physical Signals/Sinks/PS Terminator
  PS Terminator1 : fl_lib/Physical Signals/Sinks/PS Terminator
  Panel Revolute : sm_lib/Joints/Revolute Joint  JointMode=Normal  CompositeWrenchDir=FollowerOnBase  CompositeWrenchFrame=BaseFrame  SenseConstraintForce=off  SenseConstraintTorque=off  SenseTotalForce=off  SenseTotalTorque=off  PositionTargetSpecify=on  PositionTargetPriority=High  PositionTargetValue=panelrevolute.q0  PositionTargetValueUnits=deg  VelocityTargetSpecify=off  VelocityTargetPriority=High  VelocityTargetValue=0  VelocityTargetValueUnits=deg/s  EquilibriumPosition=0  EquilibriumPositionUnits=deg  SpringStiffness=0  SpringStiffnessUnits=N*m/deg  DampingCoefficient=0  DampingCoefficientUnits=N*m/(deg/s)  LowerLimitSpecify=off  LowerLimitBound=-90  LowerLimitBoundUnits=deg  LowerLimitStiffness=1e4  LowerLimitStiffnessUnits=N*m/deg  LowerLimitDamping=10  LowerLimitDampingUnits=N*m/(deg/s)  LowerLimitTransitionRegionWidth=0.1  LowerLimitTransitionRegionWidthUnits=deg  UpperLimitSpecify=off  UpperLimitBound=90  UpperLimitBoundUnits=deg  UpperLimitStiffness=1e4  UpperLimitStiffnessUnits=N*m/deg  UpperLimitDamping=10  UpperLimitDampingUnits=N*m/(deg/s)  UpperLimitTransitionRegionWidth=0.1  UpperLimitTransitionRegionWidthUnits=deg  TorqueActuationMode=ComputedTorque  MotionActuationMode=InputMotion  SensePosition=off  SenseVelocity=off  SenseAcceleration=off  SenseTorqueForce=off  SenseLowerLimitTorqueForce=off  SenseUpperLimitTorqueForce=off
  Slew Drive : WormAndGearConstraintLibrary/Slew Drive  wormLeadAngle=slewdrive.wormLeadAngle  wormLength=slewdrive.wormLength  gearOuterRadius=slewdrive.gearOuterRadius  gearInnerRadius=slewdrive.gearInnerRadius  gearExposedRadius=slewdrive.gearExposedRadius  ratio=slewdrive.ratio  housingThickness=slewdrive.housingThickness  bWormRevolute=slewdrive.wormRevoluteDamping  wormRho=slewdrive.wormDensity  gearRho=slewdrive.gearDensity  housingRho=slewdrive.housingDensity  wormColor=slewdrive.wormColor  gearColor=slewdrive.gearColor  housingColor=slewdrive.housingColor  housingOpacity=slewdrive.housingOpacity
      settings: LibrarySourceBlock=sm_solar_tracker_lib/Slew Drive
  Solar Panel Assembly : Subsystem
      mask Display:
      | image(fullfile('WormAndGearConstraintSupport','Images','SolarPanel.png'));
      | port_label('lconn',1,'H');
  Support : WormAndGearConstraintLibrary/Support  columnRadius=support.columnRadius  columnThickness=support.columnThickness  columnHeight=support.columnHeight  baseWidth=support.baseWidth  baseThickness=support.baseThickness  rho=support.density  color=support.color
      settings: LibrarySourceBlock=sm_solar_tracker_lib/Support
  B : PMIOPort  Side=Left
  y : PMIOPort  Port=2  Side=Left
  p : PMIOPort  Port=3  Side=Left
  connections:
  PS Terminator1/LConn1 -- Slew Drive/RConn3
  Panel Revolute/RConn1 -- Solar Panel Assembly/LConn1
  Panel Revolute/LConn2 -- p/RConn1
  Slew Drive/LConn2 -- y/RConn1
  PS Terminator/LConn1 -- Slew Drive/RConn2
  Panel Revolute/LConn1 -- Drive Connection/RConn1
  Drive Connection/LConn1 -- Slew Drive/RConn1
  Support/RConn1 -- Slew Drive/LConn1
  Support/LConn1 -- B/RConn1

== system Solar_Tracker_Model_Dual_axis/Subsystem/Solar Array/Solar Tracker3 ==
  Drive Connection : WormAndGearConstraintLibrary/Drive Connection  connRadius=driveconn.connectionRadius  connThickness=driveconn.connectionThickness  connLength=driveconn.connectionLength  bracketWidth=driveconn.bracketWidthHeight  bracketThickness=driveconn.bracketThickness  holeRadius=driveconn.holeRadius  holeOffset=driveconn.holeOffset  baseThickness=driveconn.baseThickness  rho=driveconn.density  color=driveconn.color
      settings: LibrarySourceBlock=sm_solar_tracker_lib/Drive Connection
  Panel Revolute : sm_lib/Joints/Revolute Joint  JointMode=Normal  CompositeWrenchDir=FollowerOnBase  CompositeWrenchFrame=BaseFrame  SenseConstraintForce=off  SenseConstraintTorque=off  SenseTotalForce=off  SenseTotalTorque=off  PositionTargetSpecify=on  PositionTargetPriority=High  PositionTargetValue=panelrevolute.q0  PositionTargetValueUnits=deg  VelocityTargetSpecify=off  VelocityTargetPriority=High  VelocityTargetValue=0  VelocityTargetValueUnits=deg/s  EquilibriumPosition=0  EquilibriumPositionUnits=deg  SpringStiffness=0  SpringStiffnessUnits=N*m/deg  DampingCoefficient=0  DampingCoefficientUnits=N*m/(deg/s)  LowerLimitSpecify=off  LowerLimitBound=-90  LowerLimitBoundUnits=deg  LowerLimitStiffness=1e4  LowerLimitStiffnessUnits=N*m/deg  LowerLimitDamping=10  LowerLimitDampingUnits=N*m/(deg/s)  LowerLimitTransitionRegionWidth=0.1  LowerLimitTransitionRegionWidthUnits=deg  UpperLimitSpecify=off  UpperLimitBound=90  UpperLimitBoundUnits=deg  UpperLimitStiffness=1e4  UpperLimitStiffnessUnits=N*m/deg  UpperLimitDamping=10  UpperLimitDampingUnits=N*m/(deg/s)  UpperLimitTransitionRegionWidth=0.1  UpperLimitTransitionRegionWidthUnits=deg  TorqueActuationMode=ComputedTorque  MotionActuationMode=InputMotion  SensePosition=off  SenseVelocity=off  SenseAcceleration=off  SenseTorqueForce=off  SenseLowerLimitTorqueForce=off  SenseUpperLimitTorqueForce=off
  Slew Drive : WormAndGearConstraintLibrary/Slew Drive  wormLeadAngle=slewdrive.wormLeadAngle  wormLength=slewdrive.wormLength  gearOuterRadius=slewdrive.gearOuterRadius  gearInnerRadius=slewdrive.gearInnerRadius  gearExposedRadius=slewdrive.gearExposedRadius  ratio=slewdrive.ratio  housingThickness=slewdrive.housingThickness  bWormRevolute=slewdrive.wormRevoluteDamping  wormRho=slewdrive.wormDensity  gearRho=slewdrive.gearDensity  housingRho=slewdrive.housingDensity  wormColor=slewdrive.wormColor  gearColor=slewdrive.gearColor  housingColor=slewdrive.housingColor  housingOpacity=slewdrive.housingOpacity
      settings: LibrarySourceBlock=sm_solar_tracker_lib/Slew Drive
  Solar Panel Assembly : Subsystem
      mask Display:
      | image(fullfile('WormAndGearConstraintSupport','Images','SolarPanel.png'));
      | port_label('lconn',1,'H');
  Support : WormAndGearConstraintLibrary/Support  columnRadius=support.columnRadius  columnThickness=support.columnThickness  columnHeight=support.columnHeight  baseWidth=support.baseWidth  baseThickness=support.baseThickness  rho=support.density  color=support.color
      settings: LibrarySourceBlock=sm_solar_tracker_lib/Support
  B : PMIOPort  Side=Left
  y : PMIOPort  Port=2  Side=Left
  p : PMIOPort  Port=3  Side=Left
  w : PMIOPort  Port=4  Side=Right
  t : PMIOPort  Port=5  Side=Right
  connections:
  Support/LConn1 -- B/RConn1
  Support/RConn1 -- Slew Drive/LConn1
  Drive Connection/LConn1 -- Slew Drive/RConn1
  Panel Revolute/LConn1 -- Drive Connection/RConn1
  w/RConn1 -- Slew Drive/RConn2
  Slew Drive/LConn2 -- y/RConn1
  Panel Revolute/LConn2 -- p/RConn1
  Panel Revolute/RConn1 -- Solar Panel Assembly/LConn1
  t/RConn1 -- Slew Drive/RConn3

== system Solar_Tracker_Model_Dual_axis/Stepper motor (1)/Controller1/Position/Algorithm and Pulse Generation ==
  note: The reference input defines the required angular position in terms of
      | the number steps. For this stepper, the step size is 1.8 degrees. Hence
      | a demand of 10 steps results in an angle change of 18 degrees.
      | The step rate is set by the Pulse Generator's Pulse rate mask parameter.
  note: Position Controller
  Reference : Inport
  IC Analog Output REV : Subsystem
  IC Analog Output Vref : Subsystem
  Logic2Volts1 : Gain  Gain=5
  Logic2Volts2 : Gain  Gain=5
  Pulse Generator : Subsystem  mask{f=20}
      mask prompts: f "Pulse rate"
  Rate Transition : RateTransition  Deterministic=off
  REV : PMIOPort  Side=Right
  Vref : PMIOPort  Port=2  Side=Right
  wires:
  Logic2Volts1/1 -> IC Analog Output Vref/1(SL)
  Pulse Generator/1(Pulse train) -> Logic2Volts1/1
  Reference/1 -> Rate Transition/1
  Logic2Volts2/1 -> IC Analog Output REV/1(SL)
  Pulse Generator/2(Pulse direction) -> Logic2Volts2/1
  Rate Transition/1 -> Pulse Generator/1(Pulse  demand)
  connections:
  Vref/RConn1 -- IC Analog Output Vref/RConn1
  REV/RConn1 -- IC Analog Output REV/RConn1

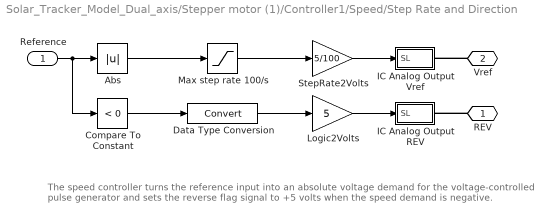
== system Solar_Tracker_Model_Dual_axis/Stepper motor (1)/Controller1/Speed/Step Rate and Direction ==
  note: The speed controller turns the reference input into an absolute voltage demand for the
      | voltage-controlled pulse generator and sets the reverse flag signal to +5 volts when the
      | speed demand is negative.
  Reference : Inport
  Abs : Abs  SaturateOnIntegerOverflow=off
  Compare To Constant : simulink/Logic and Bit Operations/Compare To Constant  relop=<  const=0  OutDataTypeStr=uint8  ZeroCross=off
  Data Type Conversion : DataTypeConversion  SaturateOnIntegerOverflow=off  RndMeth=Floor
  IC Analog Output REV : Subsystem
  IC Analog Output Vref : Subsystem
  Logic2Volts : Gain  Gain=5
  Max step rate 100/s : Saturate  UpperLimit=100  LowerLimit=0
  StepRate2Volts : Gain  Gain=5/100
  REV : PMIOPort  Side=Right
  Vref : PMIOPort  Port=2  Side=Right
  wires:
  StepRate2Volts/1 -> IC Analog Output Vref/1(SL)
  Max step rate 100/s/1 -> StepRate2Volts/1
  Data Type Conversion/1 -> Logic2Volts/1
  Compare To Constant/1 -> Data Type Conversion/1
  Reference/1 -> Compare To Constant/1, Abs/1
  Abs/1 -> Max step rate 100/s/1
  Logic2Volts/1 -> IC Analog Output REV/1(SL)
  connections:
  REV/RConn1 -- IC Analog Output REV/RConn1
  Vref/RConn1 -- IC Analog Output Vref/RConn1

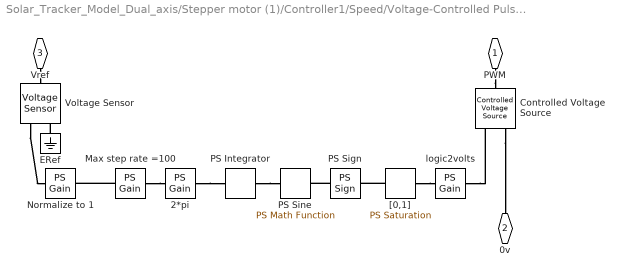
== system Solar_Tracker_Model_Dual_axis/Stepper motor (1)/Controller1/Speed/Voltage-Controlled Pulse Generator ==
  2*pi : fl_ps_legacy_lib/Legacy Physical Signals/Functions/PS Gain  gain=-2*pi
  Controlled Voltage Source : fl_lib/Electrical/Electrical Sources/Controlled Voltage Source
  ERef : fl_lib/Electrical/Electrical Elements/Electrical Reference
  Max step rate =100 : fl_ps_legacy_lib/Legacy Physical Signals/Functions/PS Gain  gain=100
  Normalize to 1 : fl_ps_legacy_lib/Legacy Physical Signals/Functions/PS Gain  gain=1/5
  PS Integrator : fl_ps_legacy_lib/Legacy Physical Signals/Linear Operators/PS Integrator  x0=0
      settings: InternalSimscapePortConfiguration="{\"Bottom\":[],\"Left\":[{\"id\":\"I\",\"label\":\"\",\"type\":\"input\"}],\"Right\":[{\"id\":\"O\",\"label\":\"\",\"type\":\"output\"}],\"Top\":[]}"
  PS Sign : fl_ps_legacy_lib/Legacy Physical Signals/Nonlinear Operators/PS Sign
      settings: InternalSimscapePortConfiguration="{\"Bottom\":[],\"Left\":[{\"id\":\"I\",\"label\":\"\",\"type\":\"input\"}],\"Right\":[{\"id\":\"O\",\"label\":\"\",\"type\":\"output\"}],\"Top\":[]}"
  PS Sine : fl_ps_legacy_lib/Legacy Physical Signals/Functions/PS Math Function  fcn_choice=1
      settings: InternalSimscapePortConfiguration="{\"Bottom\":[],\"Left\":[{\"id\":\"I\",\"label\":\"\",\"type\":\"input\"}],\"Right\":[{\"id\":\"O\",\"label\":\"\",\"type\":\"output\"}],\"Top\":[]}"
  Voltage Sensor : fl_lib/Electrical/Electrical Sensors/Voltage Sensor
  "[0,1]" : fl_ps_legacy_lib/Legacy Physical Signals/Nonlinear Operators/PS Saturation  upper_limit=1  lower_limit=0
      settings: InternalSimscapePortConfiguration="{\"Bottom\":[],\"Left\":[{\"id\":\"I\",\"label\":\"\",\"type\":\"input\"}],\"Right\":[{\"id\":\"O\",\"label\":\"\",\"type\":\"output\"}],\"Top\":[]}"
  logic2volts : fl_ps_legacy_lib/Legacy Physical Signals/Functions/PS Gain  gain=5
  PWM : PMIOPort  Side=Right
  0v : PMIOPort  Port=2  Side=Right
  Vref : PMIOPort  Port=3  Side=Left
  connections:
  PWM/RConn1 -- Controlled Voltage Source/LConn1
  Controlled Voltage Source/RConn2 -- 0v/RConn1
  Vref/RConn1 -- Voltage Sensor/LConn1
  ERef/LConn1 -- Voltage Sensor/RConn2
  Voltage Sensor/RConn1 -- Normalize to 1/LConn1
  Max step rate =100/LConn1 -- Normalize to 1/RConn1
  Max step rate =100/RConn1 -- 2*pi/LConn1
  2*pi/RConn1 -- PS Integrator/LConn1
  PS Integrator/RConn1 -- PS Sine/LConn1
  PS Sign/LConn1 -- PS Sine/RConn1
  "[0,1]"/LConn1 -- PS Sign/RConn1
  "[0,1]"/RConn1 -- logic2volts/LConn1
  logic2volts/RConn1 -- Controlled Voltage Source/RConn1

== system Solar_Tracker_Model_Dual_axis/Stepper motor (2)/Controller/Position/Algorithm and Pulse Generation ==
  note: The reference input defines the required angular position in terms of
      | the number steps. For this stepper, the step size is 1.8 degrees. Hence
      | a demand of 10 steps results in an angle change of 18 degrees.
      | The step rate is set by the Pulse Generator's Pulse rate mask parameter.
  note: Position Controller
  Reference : Inport
  IC Analog Output REV : Subsystem
  IC Analog Output Vref : Subsystem
  Logic2Volts1 : Gain  Gain=5
  Logic2Volts2 : Gain  Gain=5
  Pulse Generator : Subsystem  mask{f=20}
      mask prompts: f "Pulse rate"
  Rate Transition : RateTransition  Deterministic=off
  REV : PMIOPort  Side=Right
  Vref : PMIOPort  Port=2  Side=Right
  wires:
  Logic2Volts1/1 -> IC Analog Output Vref/1(SL)
  Pulse Generator/1(Pulse train) -> Logic2Volts1/1
  Reference/1 -> Rate Transition/1
  Logic2Volts2/1 -> IC Analog Output REV/1(SL)
  Pulse Generator/2(Pulse direction) -> Logic2Volts2/1
  Rate Transition/1 -> Pulse Generator/1(Pulse  demand)
  connections:
  Vref/RConn1 -- IC Analog Output Vref/RConn1
  REV/RConn1 -- IC Analog Output REV/RConn1
